simulink model "Func"  (R2020a)
settings: Solver=VariableStepAuto  StartTime=0.0  StopTime=100  RelTol=1e-6
undefined symbols (not defined in the file or in its folder): a1, a2, g, k, m
settings Model: Creator=faith  LastModifiedBy=faith

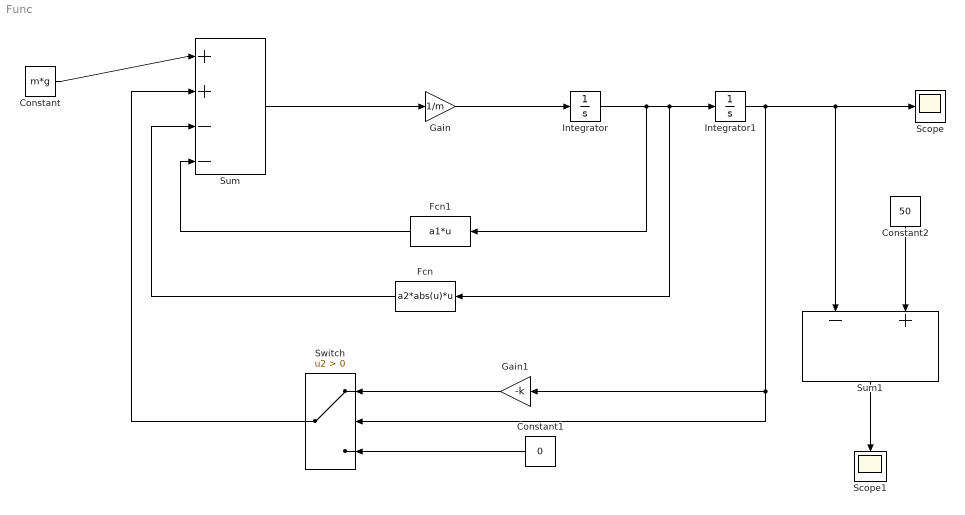
== system Func ==
  Constant : Constant  Value=m*g
  Constant1 : Constant  Value=0
  Constant2 : Constant  Value=50
  Fcn : Fcn  Expr=a2*abs(u)*u
  Fcn1 : Fcn  Expr=a1*u
  Gain : Gain  Gain=1/m
  Gain1 : Gain  Gain=-k
  Integrator : Integrator
  Integrator1 : Integrator  InitialCondition=-30
  Scope : Scope
  Scope1 : Scope
  Sum : Sum  Inputs=|++--
  Sum1 : Sum  Inputs=-+
  Switch : Switch  Criteria=u2 > Threshold
  wires:
  Constant2/1 -> Sum1/2
  Switch/1 -> Sum/2
  Integrator1/1 -> Scope/1, Sum1/1, Switch/2, Gain1/1
  Gain1/1 -> Switch/1
  Sum/1 -> Gain/1
  Constant/1 -> Sum/1
  Sum1/1 -> Scope1/1
  Constant1/1 -> Switch/3
  Fcn1/1 -> Sum/4
  Gain/1 -> Integrator/1
  Integrator/1 -> Fcn1/1, Fcn/1, Integrator1/1
  Fcn/1 -> Sum/3
